simulink model "EcoSIM3_P2_C2_WIP"  (R2014b)
settings: Solver=ode1  SolverMode=SingleTasking  StartTime=0.0  StopTime=4  FixedStep=0.01  RelTol=1e-3
PostLoadFcn:
  | %, if any(exist('dsrtsu_mdlpostloadfcn', 'file') == [2, 3, 6]), try dsrtsu_mdlpostloadfcn('Execute', bdroot); catch fprintf('Error in PostLoadFcn (dsrtsu_mdlpostloadfcn) for model "%s":\n %s\n', bdroot, lasterr); end, end,
InitFcn:
  | tic
  | %Startup_EcoSIM
undefined symbols (not defined in the file or in its folder): canChannel, Controls, DriveCycles, Driver, EM_EFF_MAP, EM_PwrLoss_MAP, EngPwr, EngSpd, EngTrq, Glbl, Overwritten_Mode, Plants, Power, sigbuilder_block, Torque, Trialmap, Veh_Dynamics
libraries: simulink x135, canmsglib x113, fl_lib x104, canlib x89, nesl_utility x56, sdl_lib x29, dspsigops x6, dspswit3 x5, dspstat3 x2, commnoisgen2 x1, dspfdesign x1
(part 17 of 21)

== system EcoSIM3_P2_C2_WIP/Powertrain/Soft_ECUs_IO/VNT Kvaser/CANTx/GMLAN/PPEI_Brake_Apply_Status ==
  GM : Inport
  Bus Selector3 : BusSelector  OutputSignals=PPEI_Brake_Apply_Status.BrkPdlPos
  CAN Pack1 : canmsglib/CAN Pack  CANdbFile=C:\Users\EcoCAR_HIL\Documents\Khanna\EcoSIM3_P1_0_PHEV_TCU\Final_DBC\GlobalAHS_anon GM CONFIDENTIAL.dbc  MsgList=PPEI_Brake_Apply_Status  MsgName=PPEI_Brake_Apply_Status  MsgIDType=Standard (11-bit identifier)  MsgIdentifier=241  MsgLength=6  SignalInfo=BrkAppSnsrHmPosLrnd$30$1$2$2$1$0$1$0$0$1$#BrkPdlChkData$40$17$2$2$1$0$1$0$0$131071$#BrkPdlInTrvPrt$2$2$2$2$1$0$1$0$0$3$#BrkPdlModTrvl$6$1$2$2$1$0$1$0$0$1$#BrkPdlModTrvlV$7$1$2$2$1$0$1$0$0$1$#BrkPdlPos$8$8$2$2$1$0$3.921570e-01$0$0$1.000000e+02$#BrkPdlPosGrad$16$8$2$1$1$0$40$0$-5120$5080$#BrkPedPosAlvRolngCnt$4$2$2$2$1$0$1$0$0$3$#BrkPedTrvlAchvd$1$1$2$2$1$0$1$0$0$1$#BrkPedTrvlAchvdV$0$1$2$2$1$0$1$0$0$1$#NotEventStat$28$2$2$2$1$0$1$0$0$3$#  NSignals=11  StartBits=str2num('[int32(30);int32(40);int32(2);int32(6);int32(7);int32(8);int32(16);int32(4);int32(1);int32(0);int32(28)]')  SignalSizes=str2num('[int32(1);int32(17);int32(2);int32(1);int32(1);int32(8);int32(8);int32(2);int32(1);int32(1);int32(2)]')  ByteOrders=str2num('[int32(2);int32(2);int32(2);int32(2);int32(2);int32(2);int32(2);int32(2);int32(2);int32(2);int32(2)]')  DataTypes=str2num('[int32(2);int32(2);int32(2);int32(2);int32(2);int32(2);int32(1);int32(2);int32(2);int32(2);int32(2)]')  MultiplexTypes=str2num('[int32(1);int32(1);int32(1);int32(1);int32(1);int32(1);int32(1);int32(1);int32(1);int32(1);int32(1)]')  MultiplexValues=str2num('[double(0);double(0);double(0);double(0);double(0);double(0);double(0);double(0);double(0);double(0);double(0)]')  Factors=str2num('[double(1);double(1);double(1);double(1);double(1);double(3.921570e-01);double(40);double(1);double(1);double(1);double(1)]')  Offsets=str2num('[double(0);double(0);double(0);double(0);double(0);double(0);double(0);double(0);double(0);double(0);double(0)]')  Minimums=str2num('[double(0);double(0);double(0);double(0);double(0);double(0);double(-5120);double(0);double(0);double(0);double(0)]')  Maximums=str2num('[double(1);double(131071);double(3);double(1);double(1);double(1.000000e+02);double(5080);double(3);double(1);double(1);double(3)]')  Remote=off
      settings: DataFormat=CANdb specified signals
  CAN Transmit2 : canlib/CAN Transmit  BlockHandle=3142.0018  DeviceMenu=Kvaser Virtual 1 (Channel 1)  Device=Kvaser Virtual 1 (Channel 1)  ObjConstructor=canChannel('Kvaser', 'Virtual 1', 1)  EnablePeriodicTransmit=off  MessagePeriod=1.000
  Ground_{1..10} (10 alike) : Ground
  Rate Transition : RateTransition
  wires:
  Ground_1/1 -> CAN Pack1/1
  Ground_5/1 -> CAN Pack1/5
  Ground_4/1 -> CAN Pack1/4
  Ground_6/1 -> CAN Pack1/7
  Ground_2/1 -> CAN Pack1/2
  Ground_3/1 -> CAN Pack1/3
  Ground_10/1 -> CAN Pack1/11
  Ground_7/1 -> CAN Pack1/8
  Ground_8/1 -> CAN Pack1/9
  Ground_9/1 -> CAN Pack1/10
  Bus Selector3/1 -> Rate Transition/1  "<BrkPdlPos>"
  GM/1 -> Bus Selector3/1
  Rate Transition/1 -> CAN Pack1/6
  CAN Pack1/1 -> CAN Transmit2/1

== system EcoSIM3_P2_C2_WIP/Powertrain/Soft_ECUs_IO/VNT Kvaser/CANTx/GMLAN/PPEI_Driven_Whl_Rotational_Stat ==
  GM : Inport
  Bus Selector2 : BusSelector  OutputSignals=PPEI_Driven_Whl_Rotational_Stat.WRSLDWhlDistPlsCntr,PPEI_Driven_Whl_Rotational_Stat.WRSRDWhlDistPlsCntr
  CAN Pack4 : canmsglib/CAN Pack  CANdbFile=C:\Users\EcoCAR_HIL\Documents\Khanna\EcoSIM3_P1_0_PHEV_TCU\Final_DBC\GlobalAHS_anon GM CONFIDENTIAL.dbc  MsgList=PPEI_Driven_Whl_Rotational_Stat  MsgName=PPEI_Driven_Whl_Rotational_Stat  MsgIDType=Standard (11-bit identifier)  MsgIdentifier=193  MsgLength=8  SignalInfo=WRSLDSeqNum$4$2$2$2$1$0$1$0$0$3$#WRSLDWhlDisTpRC$6$2$2$2$1$0$1$0$0$3$#WRSLDWhlDistPlsCntr$8$10$2$2$1$0$1$0$0$1023$#WRSLDWhlDistTmstm$24$16$2$2$1$0$1$0$0$65535$#WRSLDWhlDistVal$2$1$2$2$1$0$1$0$0$1$#WRSLDWhlRotStatRst$3$1$2$2$1$0$1$0$0$1$#WRSRDSeqNum$36$2$2$2$1$0$1$0$0$3$#WRSRDWhlDisTpRC$38$2$2$2$1$0$1$0$0$3$#WRSRDWhlDistPlsCntr$40$10$2$2$1$0$1$0$0$1023$#WRSRDWhlDistTmstm$56$16$2$2$1$0$1$0$0$65535$#WRSRDWhlDistVal$34$1$2$2$1$0$1$0$0$1$#WRSRDWhlRotStatRst$35$1$2$2$1$0$1$0$0$1$#  NSignals=12  StartBits=str2num('[int32(4);int32(6);int32(8);int32(24);int32(2);int32(3);int32(36);int32(38);int32(40);int32(56);int32(34);int32(35)]')  SignalSizes=str2num('[int32(2);int32(2);int32(10);int32(16);int32(1);int32(1);int32(2);int32(2);int32(10);int32(16);int32(1);int32(1)]')  ByteOrders=str2num('[int32(2);int32(2);int32(2);int32(2);int32(2);int32(2);int32(2);int32(2);int32(2);int32(2);int32(2);int32(2)]')  DataTypes=str2num('[int32(2);int32(2);int32(2);int32(2);int32(2);int32(2);int32(2);int32(2);int32(2);int32(2);int32(2);int32(2)]')  MultiplexTypes=str2num('[int32(1);int32(1);int32(1);int32(1);int32(1);int32(1);int32(1);int32(1);int32(1);int32(1);int32(1);int32(1)]')  MultiplexValues=str2num('[double(0);double(0);double(0);double(0);double(0);double(0);double(0);double(0);double(0);double(0);double(0);double(0)]')  Factors=str2num('[double(1);double(1);double(1);double(1);double(1);double(1);double(1);double(1);double(1);double(1);double(1);double(1)]')  Offsets=str2num('[double(0);double(0);double(0);double(0);double(0);double(0);double(0);double(0);double(0);double(0);double(0);double(0)]')  Minimums=str2num('[double(0);double(0);double(0);double(0);double(0);double(0);double(0);double(0);double(0);double(0);double(0);double(0)]')  Maximums=str2num('[double(3);double(3);double(1023);double(65535);double(1);double(1);double(3);double(3);double(1023);double(65535);double(1);double(1)]')  Remote=off
      settings: DataFormat=CANdb specified signals
  CAN Transmit2 : canlib/CAN Transmit  BlockHandle=3172.0018  DeviceMenu=Kvaser Virtual 1 (Channel 1)  Device=Kvaser Virtual 1 (Channel 1)  ObjConstructor=canChannel('Kvaser', 'Virtual 1', 1)  EnablePeriodicTransmit=off  MessagePeriod=1.000
  Ground_{50..59} (10 alike) : Ground
  Rate Transition : RateTransition
  Rate Transition1 : RateTransition
  wires:
  Bus Selector2/1 -> Rate Transition/1  "<WRSLDWhlDistPlsCntr>"
  Bus Selector2/2 -> Rate Transition1/1  "<WRSRDWhlDistPlsCntr>"
  Ground_57/1 -> CAN Pack4/10
  Ground_50/1 -> CAN Pack4/1
  Ground_59/1 -> CAN Pack4/12
  Ground_53/1 -> CAN Pack4/5
  Ground_52/1 -> CAN Pack4/4
  Ground_51/1 -> CAN Pack4/2
  Ground_54/1 -> CAN Pack4/6
  Ground_55/1 -> CAN Pack4/7
  Ground_56/1 -> CAN Pack4/8
  Ground_58/1 -> CAN Pack4/11
  GM/1 -> Bus Selector2/1
  Rate Transition/1 -> CAN Pack4/3
  Rate Transition1/1 -> CAN Pack4/9
  CAN Pack4/1 -> CAN Transmit2/1

== system EcoSIM3_P2_C2_WIP/Powertrain/Soft_ECUs_IO/VNT Kvaser/CANTx/GMLAN/PPEI_NonDrivn_Whl_Rotationl_Stat ==
  GM : Inport
  Bus Selector5 : BusSelector  OutputSignals=PPEI_NonDrivn_Whl_Rotationl_Stat.WRSLNDWhlDistPCntr,PPEI_NonDrivn_Whl_Rotationl_Stat.WRSRNDWhlDistPCntr
  CAN Pack5 : canmsglib/CAN Pack  CANdbFile=C:\Users\EcoCAR_HIL\Documents\Khanna\EcoSIM3_P1_0_PHEV_TCU\Final_DBC\GlobalAHS_anon GM CONFIDENTIAL.dbc  MsgList=PPEI_NonDrivn_Whl_Rotationl_Stat  MsgName=PPEI_NonDrivn_Whl_Rotationl_Stat  MsgIDType=Standard (11-bit identifier)  MsgIdentifier=197  MsgLength=8  SignalInfo=WRSLNDSeqNum$4$2$2$2$1$0$1$0$0$3$#WRSLNDWhlDisTpRC$6$2$2$2$1$0$1$0$0$3$#WRSLNDWhlDistPCntr$8$10$2$2$1$0$1$0$0$1023$#WRSLNDWhlDistTstm$24$16$2$2$1$0$1$0$0$65535$#WRSLNDWhlDistVal$2$1$2$2$1$0$1$0$0$1$#WRSLNDWhlRotStRst$3$1$2$2$1$0$1$0$0$1$#WRSRNDSeqNum$36$2$2$2$1$0$1$0$0$3$#WRSRNDWhlDisTpRC$38$2$2$2$1$0$1$0$0$3$#WRSRNDWhlDistPCntr$40$10$2$2$1$0$1$0$0$1023$#WRSRNDWhlDistTstm$56$16$2$2$1$0$1$0$0$65535$#WRSRNDWhlDistVal$34$1$2$2$1$0$1$0$0$1$#WRSRNDWhlRotStRst$35$1$2$2$1$0$1$0$0$1$#  NSignals=12  StartBits=str2num('[int32(4);int32(6);int32(8);int32(24);int32(2);int32(3);int32(36);int32(38);int32(40);int32(56);int32(34);int32(35)]')  SignalSizes=str2num('[int32(2);int32(2);int32(10);int32(16);int32(1);int32(1);int32(2);int32(2);int32(10);int32(16);int32(1);int32(1)]')  ByteOrders=str2num('[int32(2);int32(2);int32(2);int32(2);int32(2);int32(2);int32(2);int32(2);int32(2);int32(2);int32(2);int32(2)]')  DataTypes=str2num('[int32(2);int32(2);int32(2);int32(2);int32(2);int32(2);int32(2);int32(2);int32(2);int32(2);int32(2);int32(2)]')  MultiplexTypes=str2num('[int32(1);int32(1);int32(1);int32(1);int32(1);int32(1);int32(1);int32(1);int32(1);int32(1);int32(1);int32(1)]')  MultiplexValues=str2num('[double(0);double(0);double(0);double(0);double(0);double(0);double(0);double(0);double(0);double(0);double(0);double(0)]')  Factors=str2num('[double(1);double(1);double(1);double(1);double(1);double(1);double(1);double(1);double(1);double(1);double(1);double(1)]')  Offsets=str2num('[double(0);double(0);double(0);double(0);double(0);double(0);double(0);double(0);double(0);double(0);double(0);double(0)]')  Minimums=str2num('[double(0);double(0);double(0);double(0);double(0);double(0);double(0);double(0);double(0);double(0);double(0);double(0)]')  Maximums=str2num('[double(3);double(3);double(1023);double(65535);double(1);double(1);double(3);double(3);double(1023);double(65535);double(1);double(1)]')  Remote=off
      settings: DataFormat=CANdb specified signals
  CAN Transmit2 : canlib/CAN Transmit  BlockHandle=3205.0018  DeviceMenu=Kvaser Virtual 1 (Channel 1)  Device=Kvaser Virtual 1 (Channel 1)  ObjConstructor=canChannel('Kvaser', 'Virtual 1', 1)  EnablePeriodicTransmit=off  MessagePeriod=1.000
  Ground_{60..69} (10 alike) : Ground
  Rate Transition : RateTransition
  Rate Transition1 : RateTransition
  wires:
  Bus Selector5/2 -> Rate Transition1/1  "<WRSRNDWhlDistPCntr>"
  Bus Selector5/1 -> Rate Transition/1  "<WRSLNDWhlDistPCntr>"
  Ground_60/1 -> CAN Pack5/1
  Ground_69/1 -> CAN Pack5/12
  Ground_63/1 -> CAN Pack5/5
  Ground_61/1 -> CAN Pack5/2
  Ground_66/1 -> CAN Pack5/8
  Ground_67/1 -> CAN Pack5/10
  Ground_68/1 -> CAN Pack5/11
  Ground_65/1 -> CAN Pack5/7
  Ground_64/1 -> CAN Pack5/6
  Ground_62/1 -> CAN Pack5/4
  GM/1 -> Bus Selector5/1
  Rate Transition/1 -> CAN Pack5/3
  Rate Transition1/1 -> CAN Pack5/9
  CAN Pack5/1 -> CAN Transmit2/1

== system EcoSIM3_P2_C2_WIP/Powertrain/Soft_ECUs_IO/VNT Kvaser/CANTx/GMLAN/PPEI_Platform_General_Status ==
  GM : Inport
  Bus Selector1 : BusSelector  OutputSignals=PPEI_Platform_General_Status.SysPwrMd
  CAN Pack2 : canmsglib/CAN Pack  CANdbFile=C:\Users\EcoCAR_HIL\Documents\Khanna\EcoSIM3_P1_0_PHEV_TCU\Final_DBC\GlobalAHS_anon GM CONFIDENTIAL.dbc  MsgList=PPEI_Platform_General_Status  MsgName=PPEI_Platform_General_Status  MsgIDType=Standard (11-bit identifier)  MsgIdentifier=497  MsgLength=8  SignalInfo=ACCmpsrFldOn$63$1$2$2$1$0$1$0$0$1$#ACCompModReq$11$2$2$2$1$0$1$0$0$3$#ACCompNormLd$48$8$2$2$1$0$1.000000e-01$0$0$2.550000e+01$#ACCompNormLdV$10$1$2$2$1$0$1$0$0$1$#ACCompSysVDA$9$1$2$2$1$0$1$0$0$1$#ACCompSysVDM$60$1$2$2$1$0$1$0$0$1$#AirbgVDA$57$1$2$2$1$0$1$0$0$1$#BkupPwrModeMstrVDA$7$1$2$2$1$0$1$0$0$1$#BkupPwrModeMstrVDM$61$1$2$2$1$0$1$0$0$1$#DispMeasSys$59$1$2$2$1$0$1$0$0$1$#ElvtdIdlCstStReq$32$2$2$2$1$0$1$0$0$3$#EngOilLfRstRq$37$1$2$2$1$0$1$0$0$1$#FuelFltLfRstRqd$56$1$2$2$1$0$1$0$0$1$#ImmblzrPreRelPswdStat$8$1$2$2$1$0$1$0$0$1$#ImmblzrPreRelPswrd$24$16$2$2$1$0$1$0$0$65535$#PMMAccTrmSt$2$1$2$2$1$0$1$0$0$1$#PMMRunCrkTrmSt$3$1$2$2$1$0$1$0$0$1$#PTORSMstrEngShtReq$13$1$2$2$1$0$1$0$0$1$#PTORmStMsEngStRq$14$1$2$2$1$0$1$0$0$1$#PrkBrkSwAtv$36$1$2$2$1$0$1$0$0$1$#PrkBrkVDA$35$1$2$2$1$0$1$0$0$1$#PrkBrkVDM$62$1$2$2$1$0$1$0$0$1$#RmVehStrRq$15$1$2$2$1$0$1$0$0$1$#SIRDpl$58$1$2$2$1$0$1$0$0$1$#SysBkUpPwrMd$4$2$2$2$1$0$1$0$0$3$#SysBkupPwrMdEn$6$1$2$2$1$0$1$0$0$1$#SysPwrMd$0$2$2$2$1$0$1$0$0$3$#ThrtlPrgrsnReq$38$2$2$2$1$0$1$0$0$3$#TrStLgMdAtv$34$1$2$2$1$0$1$0$0$1$#  NSignals=29  StartBits=str2num('[int32(63);int32(11);int32(48);int32(10);int32(9);int32(60);int32(57);int32(7);int32(61);int32(59);int32(32);int32(37);int32(56);int32(8);int32(24);int32(2);int32(3);int32(13);int32(14);int32(36);int32(35);int32(62);int32(15);int32(58);int32(4);int32(6);int32(0);int32(38);int32(34)]')  SignalSizes=str2num('[int32(1);int32(2);int32(8);int32(1);int32(1);int32(1);int32(1);int32(1);int32(1);int32(1);int32(2);int32(1);int32(1);int32(1);int32(16);int32(1);int32(1);int32(1);int32(1);int32(1);int32(1);int32(1);int32(1);int32(1);int32(2);int32(1);int32(2);int32(2);int32(1)]')  ByteOrders=str2num('[int32(2);int32(2);int32(2);int32(2);int32(2);int32(2);int32(2);int32(2);int32(2);int32(2);int32(2);int32(2);int32(2);int32(2);int32(2);int32(2);int32(2);int32(2);int32(2);int32(2);int32(2);int32(2);int32(2);int32(2);int32(2);int32(2);int32(2);int32(2);int32(2)]')  DataTypes=str2num('[int32(2);int32(2);int32(2);int32(2);int32(2);int32(2);int32(2);int32(2);int32(2);int32(2);int32(2);int32(2);int32(2);int32(2);int32(2);int32(2);int32(2);int32(2);int32(2);int32(2);int32(2);int32(2);int32(2);int32(2);int32(2);int32(2);int32(2);int32(2);int32(2)]')  MultiplexTypes=str2num('[int32(1);int32(1);int32(1);int32(1);int32(1);int32(1);int32(1);int32(1);int32(1);int32(1);int32(1);int32(1);int32(1);int32(1);int32(1);int32(1);int32(1);int32(1);int32(1);int32(1);int32(1);int32(1);int32(1);int32(1);int32(1);int32(1);int32(1);int32(1);int32(1)]')  MultiplexValues=str2num('[double(0);double(0);double(0);double(0);double(0);double(0);double(0);double(0);double(0);double(0);double(0);double(0);double(0);double(0);double(0);double(0);double(0);double(0);double(0);double(0);double(0);double(0);double(0);double(0);double(0);double(0);double(0);double(0);double(0)]')  Factors=str2num('[double(1);double(1);double(1.000000e-01);double(1);double(1);double(1);double(1);double(1);double(1);double(1);double(1);double(1);double(1);double(1);double(1);double(1);double(1);double(1);double(1);double(1);double(1);double(1);double(1);double(1);double(1);double(1);double(1);double(1);double(1)]')  Offsets=str2num('[double(0);double(0);double(0);double(0);double(0);double(0);double(0);double(0);double(0);double(0);double(0);double(0);double(0);double(0);double(0);double(0);double(0);double(0);double(0);double(0);double(0);double(0);double(0);double(0);double(0);double(0);double(0);double(0);double(0)]')  Minimums=str2num('[double(0);double(0);double(0);double(0);double(0);double(0);double(0);double(0);double(0);double(0);double(0);double(0);double(0);double(0);double(0);double(0);double(0);double(0);double(0);double(0);double(0);double(0);double(0);double(0);double(0);double(0);double(0);double(0);double(0)]')  Maximums=str2num('[double(1);double(3);double(2.550000e+01);double(1);double(1);double(1);double(1);double(1);double(1);double(1);double(3);double(1);double(1);double(1);double(65535);double(1);double(1);double(1);double(1);double(1);double(1);double(1);double(1);double(1);double(3);double(1);double(3);double(3);double(1)]')  Remote=off
      settings: DataFormat=CANdb specified signals
  CAN Transmit2 : canlib/CAN Transmit  BlockHandle=3238.0018  DeviceMenu=Kvaser Virtual 1 (Channel 1)  Device=Kvaser Virtual 1 (Channel 1)  ObjConstructor=canChannel('Kvaser', 'Virtual 1', 1)  EnablePeriodicTransmit=off  MessagePeriod=1.000
  Ground_{11..38} (28 alike) : Ground
  Rate Transition : RateTransition
  wires:
  Ground_29/1 -> CAN Pack2/19
  Ground_32/1 -> CAN Pack2/22
  Ground_35/1 -> CAN Pack2/25
  Ground_11/1 -> CAN Pack2/1
  Ground_27/1 -> CAN Pack2/17
  Ground_15/1 -> CAN Pack2/5
  Ground_37/1 -> CAN Pack2/28
  Ground_13/1 -> CAN Pack2/3
  Ground_16/1 -> CAN Pack2/6
  Ground_24/1 -> CAN Pack2/14
  Ground_25/1 -> CAN Pack2/15
  Ground_14/1 -> CAN Pack2/4
  Ground_28/1 -> CAN Pack2/18
  Ground_31/1 -> CAN Pack2/21
  Ground_38/1 -> CAN Pack2/29
  Ground_21/1 -> CAN Pack2/11
  Ground_26/1 -> CAN Pack2/16
  Ground_30/1 -> CAN Pack2/20
  Ground_20/1 -> CAN Pack2/10
  Ground_17/1 -> CAN Pack2/7
  Ground_22/1 -> CAN Pack2/12
  Ground_36/1 -> CAN Pack2/26
  Ground_33/1 -> CAN Pack2/23
  Ground_18/1 -> CAN Pack2/8
  Ground_34/1 -> CAN Pack2/24
  Ground_12/1 -> CAN Pack2/2
  Ground_19/1 -> CAN Pack2/9
  Ground_23/1 -> CAN Pack2/13
  Bus Selector1/1 -> Rate Transition/1  "<SysPwrMd>"
  GM/1 -> Bus Selector1/1
  Rate Transition/1 -> CAN Pack2/27
  CAN Pack2/1 -> CAN Transmit2/1

== system EcoSIM3_P2_C2_WIP/Powertrain/Soft_ECUs_IO/VNT Kvaser/CANTx/GMLAN/PPEI_Vehicle_Speed_and_Distance ==
  GM : Inport
  Bus Selector4 : BusSelector  OutputSignals=PPEI_Vehicle_Speed_and_Distance.VehSpdAvgDrvn
  CAN Pack3 : canmsglib/CAN Pack  CANdbFile=C:\Users\EcoCAR_HIL\Documents\Khanna\EcoSIM3_P1_0_PHEV_TCU\Final_DBC\GlobalAHS_anon GM CONFIDENTIAL.dbc  MsgList=PPEI_Vehicle_Speed_and_Distance  MsgName=PPEI_Vehicle_Speed_and_Distance  MsgIDType=Standard (11-bit identifier)  MsgIdentifier=1001  MsgLength=8  SignalInfo=DistRollCntAvgDrvn$24$13$2$2$1$0$1.250000e-01$0$0$1.023875e+03$#DistRollCntAvgDrvnSrc$55$1$2$2$1$0$1$0$0$1$#DistRollCntAvgDrvnV$22$1$2$2$1$0$1$0$0$1$#DstRolCntAvNDrRstOc$53$1$2$2$1$0$1$0$0$1$#DstRolCntAvgDrnRstOc$21$1$2$2$1$0$1$0$0$1$#DstRolCntAvgNonDrvn$56$13$2$2$1$0$1.250000e-01$0$0$1.023875e+03$#DstRolCntAvgNonDrvnV$54$1$2$2$1$0$1$0$0$1$#VehSpdAvgDrvn$8$15$2$2$1$0$1.562500e-02$0$0$5.119844e+02$#VehSpdAvgDrvnSrc$23$1$2$2$1$0$1$0$0$1$#VehSpdAvgDrvnV$7$1$2$2$1$0$1$0$0$1$#VehSpdAvgNDrvn$40$15$2$2$1$0$1.562500e-02$0$0$5.119844e+02$#VehSpdAvgNDrvnV$39$1$2$2$1$0$1$0$0$1$#  NSignals=12  StartBits=str2num('[int32(24);int32(55);int32(22);int32(53);int32(21);int32(56);int32(54);int32(8);int32(23);int32(7);int32(40);int32(39)]')  SignalSizes=str2num('[int32(13);int32(1);int32(1);int32(1);int32(1);int32(13);int32(1);int32(15);int32(1);int32(1);int32(15);int32(1)]')  ByteOrders=str2num('[int32(2);int32(2);int32(2);int32(2);int32(2);int32(2);int32(2);int32(2);int32(2);int32(2);int32(2);int32(2)]')  DataTypes=str2num('[int32(2);int32(2);int32(2);int32(2);int32(2);int32(2);int32(2);int32(2);int32(2);int32(2);int32(2);int32(2)]')  MultiplexTypes=str2num('[int32(1);int32(1);int32(1);int32(1);int32(1);int32(1);int32(1);int32(1);int32(1);int32(1);int32(1);int32(1)]')  MultiplexValues=str2num('[double(0);double(0);double(0);double(0);double(0);double(0);double(0);double(0);double(0);double(0);double(0);double(0)]')  Factors=str2num('[double(1.250000e-01);double(1);double(1);double(1);double(1);double(1.250000e-01);double(1);double(1.562500e-02);double(1);double(1);double(1.562500e-02);double(1)]')  Offsets=str2num('[double(0);double(0);double(0);double(0);double(0);double(0);double(0);double(0);double(0);double(0);double(0);double(0)]')  Minimums=str2num('[double(0);double(0);double(0);double(0);double(0);double(0);double(0);double(0);double(0);double(0);double(0);double(0)]')  Maximums=str2num('[double(1.023875e+03);double(1);double(1);double(1);double(1);double(1.023875e+03);double(1);double(5.119844e+02);double(1);double(1);double(5.119844e+02);double(1)]')  Remote=off
      settings: DataFormat=CANdb specified signals
  CAN Transmit2 : canlib/CAN Transmit  BlockHandle=3304.0018  DeviceMenu=Kvaser Virtual 1 (Channel 1)  Device=Kvaser Virtual 1 (Channel 1)  ObjConstructor=canChannel('Kvaser', 'Virtual 1', 1)  EnablePeriodicTransmit=off  MessagePeriod=1.000
  Ground_{39..49} (11 alike) : Ground
  Rate Transition : RateTransition
  wires:
  Ground_47/1 -> CAN Pack3/10
  Ground_45/1 -> CAN Pack3/7
  Ground_44/1 -> CAN Pack3/6
  Ground_46/1 -> CAN Pack3/9
  Ground_49/1 -> CAN Pack3/12
  Ground_48/1 -> CAN Pack3/11
  Ground_42/1 -> CAN Pack3/4
  Ground_40/1 -> CAN Pack3/2
  Ground_39/1 -> CAN Pack3/1
  Ground_43/1 -> CAN Pack3/5
  Ground_41/1 -> CAN Pack3/3
  Bus Selector4/1 -> Rate Transition/1  "<VehSpdAvgDrvn>"
  GM/1 -> Bus Selector4/1
  Rate Transition/1 -> CAN Pack3/8
  CAN Pack3/1 -> CAN Transmit2/1

== system EcoSIM3_P2_C2_WIP/Powertrain/Soft_ECUs_IO/VNT Vector/CANTx/BAS/Status_1 ==
  In1 : Inport
  Bus Selector5 : BusSelector  OutputSignals=Status_1.BAS_Speed_rad_per_s,Status_1.BAS_Torque_Out_Nm
  CAN Pack5 : canmsglib/CAN Pack  CANdbFile=C:\Box Sync\EcoCAR 3\SMS\EcoSIM3_P2_C2\MIL\Final_DBC\InfineonInverter.dbc  MsgList=Status_1  MsgName=Status_1  MsgIDType=Standard (11-bit identifier)  MsgIdentifier=257  MsgLength=8  SignalInfo=Checksum3$0$8$1$2$1$0$1$0$-Inf$Inf$#CoolingReq$55$1$1$2$1$0$1$0$0$1$#Counter3$8$8$1$2$1$0$1$0$0$15$#ErrorInfo$48$2$1$2$1$0$1$0$0$3$#PowerRed$50$4$1$2$1$0$1$0$0$15$#ReadyHV$54$1$1$2$1$0$1$0$0$1$#RegAtLimit$56$1$1$2$1$0$1$0$0$1$#Reserved4$59$1$1$2$1$0$1$0$0$1$#SetLimitsOk$57$1$1$2$1$0$1$0$0$1$#SetValuesOk$58$1$1$2$1$0$1$0$0$1$#Speed$32$16$1$1$1$0$5.000000e-01$0$-16384$1.638350e+04$#StatusMode$60$4$1$2$1$0$1$0$0$15$#Torque_Normalized$16$16$1$1$1$0$3.051758e-05$0$-1$9.999695e-01$#  NSignals=13  StartBits=str2num('[int32(0);int32(55);int32(8);int32(48);int32(50);int32(54);int32(56);int32(59);int32(57);int32(58);int32(32);int32(60);int32(16)]')  SignalSizes=str2num('[int32(8);int32(1);int32(8);int32(2);int32(4);int32(1);int32(1);int32(1);int32(1);int32(1);int32(16);int32(4);int32(16)]')  ByteOrders=str2num('[int32(1);int32(1);int32(1);int32(1);int32(1);int32(1);int32(1);int32(1);int32(1);int32(1);int32(1);int32(1);int32(1)]')  DataTypes=str2num('[int32(2);int32(2);int32(2);int32(2);int32(2);int32(2);int32(2);int32(2);int32(2);int32(2);int32(1);int32(2);int32(1)]')  MultiplexTypes=str2num('[int32(1);int32(1);int32(1);int32(1);int32(1);int32(1);int32(1);int32(1);int32(1);int32(1);int32(1);int32(1);int32(1)]')  MultiplexValues=str2num('[double(0);double(0);double(0);double(0);double(0);double(0);double(0);double(0);double(0);double(0);double(0);double(0);double(0)]')  Factors=str2num('[double(1);double(1);double(1);double(1);double(1);double(1);double(1);double(1);double(1);double(1);double(5.000000e-01);double(1);double(3.051758e-05)]')  Offsets=str2num('[double(0);double(0);double(0);double(0);double(0);double(0);double(0);double(0);double(0);double(0);double(0);double(0);double(0)]')  Minimums=str2num('[double(-Inf);double(0);double(0);double(0);double(0);double(0);double(0);double(0);double(0);double(0);double(-16384);double(0);double(-1)]')  Maximums=str2num('[double(Inf);double(1);double(15);double(3);double(15);double(1);double(1);double(1);double(1);double(1);double(1.638350e+04);double(15);double(9.999695e-01)]')  Remote=off
      settings: DataFormat=CANdb specified signals
  Ground_{16..26} (11 alike) : Ground
  Rate Transition : RateTransition
  Rate Transition1 : RateTransition
  Out1 : Outport
  wires:
  In1/1 -> Bus Selector5/1
  CAN Pack5/1 -> Out1/1
  Ground_24/1 -> CAN Pack5/9
  Ground_26/1 -> CAN Pack5/12
  Bus Selector5/2 -> Rate Transition1/1  "<BAS_Torque_Out_Nm>"
  Ground_22/1 -> CAN Pack5/7
  Ground_19/1 -> CAN Pack5/4
  Bus Selector5/1 -> Rate Transition/1  "<BAS_Speed_rad_per_s>"
  Ground_23/1 -> CAN Pack5/8
  Ground_18/1 -> CAN Pack5/3
  Ground_20/1 -> CAN Pack5/5
  Ground_21/1 -> CAN Pack5/6
  Ground_25/1 -> CAN Pack5/10
  Ground_17/1 -> CAN Pack5/2
  Ground_16/1 -> CAN Pack5/1
  Rate Transition/1 -> CAN Pack5/11
  Rate Transition1/1 -> CAN Pack5/13

== system EcoSIM3_P2_C2_WIP/Powertrain/Soft_ECUs_IO/VNT Vector/CANTx/BAS/Status_2 ==
  In1 : Inport
  Bus Selector1 : BusSelector  OutputSignals=Status_2.Fault_U,Status_2.Fault_V,Status_2.Fault_W
  CAN Pack1 : canmsglib/CAN Pack  CANdbFile=C:\Box Sync\EcoCAR 3\SMS\EcoSIM3_P2_C2\MIL\Final_DBC\InfineonInverter.dbc  MsgList=Status_2  MsgName=Status_2  MsgIDType=Standard (11-bit identifier)  MsgIdentifier=273  MsgLength=8  SignalInfo=Checksum4$0$8$1$2$1$0$1$0$-Inf$Inf$#Counter4$8$4$1$2$1$0$1$0$0$15$#CurrentD_Limit$32$16$1$1$3$7$3.125000e-02$0$-1024$1.023969e+03$#CurrentD_Reference$32$16$1$1$3$9$3.125000e-02$0$-1024$1.023969e+03$#CurrentQ_Limit$32$16$1$1$3$6$3.125000e-02$0$-1024$1.023969e+03$#CurrentQ_Reference$32$16$1$1$3$8$3.125000e-02$0$-1024$1.023969e+03$#FaultU$13$1$1$2$1$0$1$0$0$1$#FaultV$14$1$1$2$1$0$1$0$0$1$#FaultW$15$1$1$2$1$0$1$0$0$1$#MultiplexCode$48$16$1$2$2$0$1$0$0$65535$#PhaseU_IGBT_Temp$32$16$1$1$3$3$7.812500e-03$0$-256$2.559922e+02$#PhaseV_IGBT_Temp$32$16$1$1$3$4$7.812500e-03$0$-256$2.559922e+02$#PhaseW_IGBT_Temp$32$16$1$1$3$5$7.812500e-03$0$-256$2.559922e+02$#RehabilitationReq$12$1$1$2$1$0$1$0$0$1$#Software_Version$32$16$1$2$3$0$1$0$0$65535$#Speed_Command$32$16$1$1$3$1$5.000000e-01$0$-16384$1.638350e+04$#Stator_Temperature$32$16$1$1$3$2$7.812500e-03$0$-256$2.559922e+02$#VoltageDC$16$16$1$1$1$0$3.125000e-02$0$-1024$1.023969e+03$#  NSignals=18  StartBits=str2num('[int32(0);int32(8);int32(32);int32(32);int32(32);int32(32);int32(13);int32(14);int32(15);int32(48);int32(32);int32(32);int32(32);int32(12);int32(32);int32(32);int32(32);int32(16)]')  SignalSizes=str2num('[int32(8);int32(4);int32(16);int32(16);int32(16);int32(16);int32(1);int32(1);int32(1);int32(16);int32(16);int32(16);int32(16);int32(1);int32(16);int32(16);int32(16);int32(16)]')  ByteOrders=str2num('[int32(1);int32(1);int32(1);int32(1);int32(1);int32(1);int32(1);int32(1);int32(1);int32(1);int32(1);int32(1);int32(1);int32(1);int32(1);int32(1);int32(1);int32(1)]')  DataTypes=str2num('[int32(2);int32(2);int32(1);int32(1);int32(1);int32(1);int32(2);int32(2);int32(2);int32(2);int32(1);int32(1);int32(1);int32(2);int32(2);int32(1);int32(1);int32(1)]')  MultiplexTypes=str2num('[int32(1);int32(1);int32(3);int32(3);int32(3);int32(3);int32(1);int32(1);int32(1);int32(2);int32(3);int32(3);int32(3);int32(1);int32(3);int32(3);int32(3);int32(1)]')  MultiplexValues=str2num('[double(0);double(0);double(7);double(9);double(6);double(8);double(0);double(0);double(0);double(0);double(3);double(4);double(5);double(0);double(0);double(1);double(2);double(0)]')  Factors=str2num('[double(1);double(1);double(3.125000e-02);double(3.125000e-02);double(3.125000e-02);double(3.125000e-02);double(1);double(1);double(1);double(1);double(7.812500e-03);double(7.812500e-03);double(7.812500e-03);double(1);double(1);double(5.000000e-01);double(7.812500e-03);double(3.125000e-02)]')  Offsets=str2num('[double(0);double(0);double(0);double(0);double(0);double(0);double(0);double(0);double(0);double(0);double(0);double(0);double(0);double(0);double(0);double(0);double(0);double(0)]')  Minimums=str2num('[double(-Inf);double(0);double(-1024);double(-1024);double(-1024);double(-1024);double(0);double(0);double(0);double(0);double(-256);double(-256);double(-256);double(0);double(0);double(-16384);double(-256);double(-1024)]')  Maximums=str2num('[double(Inf);double(15);double(1.023969e+03);double(1.023969e+03);double(1.023969e+03);double(1.023969e+03);double(1);double(1);double(1);double(65535);double(2.559922e+02);double(2.559922e+02);double(2.559922e+02);double(1);double(65535);double(1.638350e+04);double(2.559922e+02);double(1.023969e+03)]')  Remote=off
      settings: DataFormat=CANdb specified signals
  Ground_{1..15} (15 alike) : Ground
  Rate Transition1 : RateTransition
  Rate Transition2 : RateTransition
  Rate Transition3 : RateTransition
  Out1 : Outport
  wires:
  Ground_9/1 -> CAN Pack1/12
  Bus Selector1/3 -> Rate Transition3/1  "<Fault_W>"
  Ground_1/1 -> CAN Pack1/1
  Ground_6/1 -> CAN Pack1/6
  In1/1 -> Bus Selector1/1
  CAN Pack1/1 -> Out1/1
  Bus Selector1/2 -> Rate Transition2/1  "<Fault_V>"
  Ground_2/1 -> CAN Pack1/2
  Ground_14/1 -> CAN Pack1/17
  Ground_4/1 -> CAN Pack1/4
  Ground_12/1 -> CAN Pack1/15
  Bus Selector1/1 -> Rate Transition1/1  "<Fault_U>"
  Ground_11/1 -> CAN Pack1/14
  Ground_3/1 -> CAN Pack1/3
  Ground_10/1 -> CAN Pack1/13
  Ground_13/1 -> CAN Pack1/16
  Ground_7/1 -> CAN Pack1/10
  Ground_8/1 -> CAN Pack1/11
  Ground_5/1 -> CAN Pack1/5
  Ground_15/1 -> CAN Pack1/18
  Rate Transition1/1 -> CAN Pack1/7
  Rate Transition2/1 -> CAN Pack1/8
  Rate Transition3/1 -> CAN Pack1/9

== system EcoSIM3_P2_C2_WIP/Powertrain/Soft_ECUs_IO/VNT Vector/CANTx/EM/M160_Temperature_Set_1 ==
  EM : Inport
  Bus Selector5 : BusSelector  OutputSignals=M160_Temperature_Set_1.Module_A,M160_Temperature_Set_1.Module_B,M160_Temperature_Set_1.Module_C,M160_Temperature_Set_1.Gate_Driver_Board
  CAN Pack3 : canmsglib/CAN Pack  CANdbFile=C:\Users\EcoCAR_HIL\Documents\Khanna\EcoSIM3_P1_0_PHEV_TCU\Final_DBC\20160113 RMS PM CAN DB.dbc  MsgList=M160_Temperature_Set_1  MsgName=M160_Temperature_Set_1  MsgIDType=Standard (11-bit identifier)  MsgIdentifier=160  MsgLength=8  SignalInfo=D1_Module_A$0$16$1$1$1$0$1.000000e-01$0$-3.276800e+03$3.276700e+03$#D2_Module_B$16$16$1$1$1$0$1.000000e-01$0$-3.276800e+03$3.276700e+03$#D3_Module_C$32$16$1$1$1$0$1.000000e-01$0$-3.276800e+03$3.276700e+03$#D4_Gate_Driver_Board$48$16$1$1$1$0$1.000000e-01$0$-3.276800e+03$3.276700e+03$#  NSignals=4  StartBits=str2num('[int32(0);int32(16);int32(32);int32(48)]')  SignalSizes=str2num('[int32(16);int32(16);int32(16);int32(16)]')  ByteOrders=str2num('[int32(1);int32(1);int32(1);int32(1)]')  DataTypes=str2num('[int32(1);int32(1);int32(1);int32(1)]')  MultiplexTypes=str2num('[int32(1);int32(1);int32(1);int32(1)]')  MultiplexValues=str2num('[double(0);double(0);double(0);double(0)]')  Factors=str2num('[double(1.000000e-01);double(1.000000e-01);double(1.000000e-01);double(1.000000e-01)]')  Offsets=str2num('[double(0);double(0);double(0);double(0)]')  Minimums=str2num('[double(-3.276800e+03);double(-3.276800e+03);double(-3.276800e+03);double(-3.276800e+03)]')  Maximums=str2num('[double(3.276700e+03);double(3.276700e+03);double(3.276700e+03);double(3.276700e+03)]')  Remote=off
      settings: DataFormat=CANdb specified signals
  Rate Transition{,1..3} (4 alike) : RateTransition
  Out1 : Outport
  wires:
  Bus Selector5/2 -> Rate Transition3/1  "<Module_B>"
  Bus Selector5/4 -> Rate Transition1/1  "<Gate_Driver_Board>"
  Bus Selector5/1 -> Rate Transition/1  "<Module_A>"
  Bus Selector5/3 -> Rate Transition2/1  "<Module_C>"
  EM/1 -> Bus Selector5/1
  Rate Transition/1 -> CAN Pack3/1
  Rate Transition1/1 -> CAN Pack3/4
  Rate Transition2/1 -> CAN Pack3/3
  Rate Transition3/1 -> CAN Pack3/2
  CAN Pack3/1 -> Out1/1

== system EcoSIM3_P2_C2_WIP/Powertrain/Soft_ECUs_IO/VNT Vector/CANTx/EM/M161_Temperature_Set_2 ==
  EM : Inport
  Bus Selector6 : BusSelector  OutputSignals=M161_Temperature_Set_2.Control_Board_Temperature
  CAN Pack5 : canmsglib/CAN Pack  CANdbFile=C:\Users\EcoCAR_HIL\Documents\Khanna\EcoSIM3_P1_0_PHEV_TCU\Final_DBC\20160113 RMS PM CAN DB.dbc  MsgList=M161_Temperature_Set_2  MsgName=M161_Temperature_Set_2  MsgIDType=Standard (11-bit identifier)  MsgIdentifier=161  MsgLength=8  SignalInfo=D1_Control_Board_Temperature$0$16$1$1$1$0$1.000000e-01$0$-3.276800e+03$3.276700e+03$#D2_RTD1_Temperature$16$16$1$1$1$0$1.000000e-01$0$-3.276800e+03$3.276700e+03$#D3_RTD2_Temperature$32$16$1$1$1$0$1.000000e-01$0$-3.276800e+03$3.276700e+03$#D4_RTD3_Temperature$48$16$1$1$1$0$1.000000e-01$0$-3.276800e+03$3.276700e+03$#  NSignals=4  StartBits=str2num('[int32(0);int32(16);int32(32);int32(48)]')  SignalSizes=str2num('[int32(16);int32(16);int32(16);int32(16)]')  ByteOrders=str2num('[int32(1);int32(1);int32(1);int32(1)]')  DataTypes=str2num('[int32(1);int32(1);int32(1);int32(1)]')  MultiplexTypes=str2num('[int32(1);int32(1);int32(1);int32(1)]')  MultiplexValues=str2num('[double(0);double(0);double(0);double(0)]')  Factors=str2num('[double(1.000000e-01);double(1.000000e-01);double(1.000000e-01);double(1.000000e-01)]')  Offsets=str2num('[double(0);double(0);double(0);double(0)]')  Minimums=str2num('[double(-3.276800e+03);double(-3.276800e+03);double(-3.276800e+03);double(-3.276800e+03)]')  Maximums=str2num('[double(3.276700e+03);double(3.276700e+03);double(3.276700e+03);double(3.276700e+03)]')  Remote=off
      settings: DataFormat=CANdb specified signals
  Ground5 : Ground
  Rate Transition : RateTransition
  Out1 : Outport
  wires:
  Bus Selector6/1 -> Rate Transition/1  "<Control_Board_Temperature>"
  Ground5/1 -> CAN Pack5/3, CAN Pack5/2, CAN Pack5/4
  EM/1 -> Bus Selector6/1
  Rate Transition/1 -> CAN Pack5/1
  CAN Pack5/1 -> Out1/1

== system EcoSIM3_P2_C2_WIP/Powertrain/Soft_ECUs_IO/VNT Vector/CANTx/EM/M162_Temperature_Set_3 ==
  EM : Inport
  Bus Selector7 : BusSelector  OutputSignals=M162_Temperature_Set_3.Motor_Temperature
  CAN Pack6 : canmsglib/CAN Pack  CANdbFile=C:\Users\EcoCAR_HIL\Documents\Khanna\EcoSIM3_P1_0_PHEV_TCU\Final_DBC\20160113 RMS PM CAN DB.dbc  MsgList=M162_Temperature_Set_3  MsgName=M162_Temperature_Set_3  MsgIDType=Standard (11-bit identifier)  MsgIdentifier=162  MsgLength=8  SignalInfo=D1_RTD4_Temperature$0$16$1$1$1$0$1.000000e-01$0$-3.276800e+03$3.276700e+03$#D2_RTD5_Temperature$16$16$1$1$1$0$1.000000e-01$0$-3.276800e+03$3.276700e+03$#D3_Motor_Temperature$32$16$1$1$1$0$1.000000e-01$0$-3.276800e+03$3.276700e+03$#D4_Torque_Shudder$48$16$1$1$1$0$1.000000e-01$0$-3.276800e+03$3.276700e+03$#  NSignals=4  StartBits=str2num('[int32(0);int32(16);int32(32);int32(48)]')  SignalSizes=str2num('[int32(16);int32(16);int32(16);int32(16)]')  ByteOrders=str2num('[int32(1);int32(1);int32(1);int32(1)]')  DataTypes=str2num('[int32(1);int32(1);int32(1);int32(1)]')  MultiplexTypes=str2num('[int32(1);int32(1);int32(1);int32(1)]')  MultiplexValues=str2num('[double(0);double(0);double(0);double(0)]')  Factors=str2num('[double(1.000000e-01);double(1.000000e-01);double(1.000000e-01);double(1.000000e-01)]')  Offsets=str2num('[double(0);double(0);double(0);double(0)]')  Minimums=str2num('[double(-3.276800e+03);double(-3.276800e+03);double(-3.276800e+03);double(-3.276800e+03)]')  Maximums=str2num('[double(3.276700e+03);double(3.276700e+03);double(3.276700e+03);double(3.276700e+03)]')  Remote=off
      settings: DataFormat=CANdb specified signals
  Ground6 : Ground
  Rate Transition : RateTransition
  Out1 : Outport
  wires:
  Ground6/1 -> CAN Pack6/1, CAN Pack6/2, CAN Pack6/4
  Bus Selector7/1 -> Rate Transition/1  "<Motor_Temperature>"
  EM/1 -> Bus Selector7/1
  Rate Transition/1 -> CAN Pack6/3
  CAN Pack6/1 -> Out1/1

== system EcoSIM3_P2_C2_WIP/Powertrain/Soft_ECUs_IO/VNT Vector/CANTx/EM/M165_Motor_Position_Info ==
  EM : Inport
  Bus Selector1 : BusSelector  OutputSignals=M165_Motor_Position_Info.Motor_Speed
  CAN Pack1 : canmsglib/CAN Pack  CANdbFile=C:\Users\EcoCAR_HIL\Documents\Khanna\EcoSIM3_P1_0_PHEV_TCU\Final_DBC\20160113 RMS PM CAN DB.dbc  MsgList=M165_Motor_Position_Info  MsgName=M165_Motor_Position_Info  MsgIDType=Standard (11-bit identifier)  MsgIdentifier=165  MsgLength=8  SignalInfo=D1_Motor_Angle_Electrical$0$16$1$2$1$0$1.000000e-01$0$0$6.553500e+03$#D2_Motor_Speed$16$16$1$1$1$0$1$0$-32768$32767$#D3_Electrical_Output_Frequency$32$16$1$1$1$0$1.000000e-01$0$-3.276800e+03$3.276700e+03$#D4_Delta_Resolver_Filtered$48$16$1$1$1$0$1.000000e-01$0$-3.276800e+03$3.276700e+03$#  NSignals=4  StartBits=str2num('[int32(0);int32(16);int32(32);int32(48)]')  SignalSizes=str2num('[int32(16);int32(16);int32(16);int32(16)]')  ByteOrders=str2num('[int32(1);int32(1);int32(1);int32(1)]')  DataTypes=str2num('[int32(2);int32(1);int32(1);int32(1)]')  MultiplexTypes=str2num('[int32(1);int32(1);int32(1);int32(1)]')  MultiplexValues=str2num('[double(0);double(0);double(0);double(0)]')  Factors=str2num('[double(1.000000e-01);double(1);double(1.000000e-01);double(1.000000e-01)]')  Offsets=str2num('[double(0);double(0);double(0);double(0)]')  Minimums=str2num('[double(0);double(-32768);double(-3.276800e+03);double(-3.276800e+03)]')  Maximums=str2num('[double(6.553500e+03);double(32767);double(3.276700e+03);double(3.276700e+03)]')  Remote=off
      settings: DataFormat=CANdb specified signals
  Ground1 : Ground
  Rate Transition : RateTransition
  Out1 : Outport
  wires:
  Bus Selector1/1 -> Rate Transition/1  "<Motor_Speed>"
  CAN Pack1/1 -> Out1/1
  Ground1/1 -> CAN Pack1/1, CAN Pack1/3, CAN Pack1/4
  EM/1 -> Bus Selector1/1
  Rate Transition/1 -> CAN Pack1/2

== system EcoSIM3_P2_C2_WIP/Powertrain/Soft_ECUs_IO/VNT Vector/CANTx/EM/M170_Internal_States ==
  EM : Inport
  Bus Selector3 : BusSelector  OutputSignals=M170_Internal_States.VSM_State,M170_Internal_States.Inverter_Enable_Lockout,M170_Internal_States.Direction_Command_Feedback
  CAN Pack4 : canmsglib/CAN Pack  CANdbFile=C:\Users\EcoCAR_HIL\Documents\Khanna\EcoSIM3_P1_0_PHEV_TCU\Final_DBC\20160113 RMS PM CAN DB.dbc  MsgList=M170_Internal_States  MsgName=M170_Internal_States  MsgIDType=Standard (11-bit identifier)  MsgIdentifier=170  MsgLength=8  SignalInfo=D1_VSM_State$0$16$1$2$1$0$1$0$0$15$#D2_Inverter_State$16$8$1$2$1$0$1$0$0$255$#D3_Relay_1_Status$24$1$1$2$1$0$1$0$0$1$#D3_Relay_2_Status$25$1$1$2$1$0$1$0$0$1$#D3_Relay_3_Status$26$1$1$2$1$0$1$0$0$1$#D3_Relay_4_Status$27$1$1$2$1$0$1$0$0$1$#D3_Relay_5_Status$28$1$1$2$1$0$1$0$-Inf$Inf$#D3_Relay_6_Status$29$1$1$2$1$0$1$0$-Inf$Inf$#D4_Inverter_Discharge_State$37$3$1$2$1$0$1$0$0$7$#D4_Inverter_Run_Mode$32$1$1$2$1$0$1$0$0$1$#D5_Inverter_Command_Mode$40$1$1$2$1$0$1$0$0$1$#D6_Inverter_Enable_Lockout$55$1$1$2$1$0$1$0$0$1$#D6_Inverter_Enable_State$48$1$1$2$1$0$1$0$0$1$#D7_Direction_Command$56$8$1$2$1$0$1$0$0$1$#  NSignals=14  StartBits=str2num('[int32(0);int32(16);int32(24);int32(25);int32(26);int32(27);int32(28);int32(29);int32(37);int32(32);int32(40);int32(55);int32(48);int32(56)]')  SignalSizes=str2num('[int32(16);int32(8);int32(1);int32(1);int32(1);int32(1);int32(1);int32(1);int32(3);int32(1);int32(1);int32(1);int32(1);int32(8)]')  ByteOrders=str2num('[int32(1);int32(1);int32(1);int32(1);int32(1);int32(1);int32(1);int32(1);int32(1);int32(1);int32(1);int32(1);int32(1);int32(1)]')  DataTypes=str2num('[int32(2);int32(2);int32(2);int32(2);int32(2);int32(2);int32(2);int32(2);int32(2);int32(2);int32(2);int32(2);int32(2);int32(2)]')  MultiplexTypes=str2num('[int32(1);int32(1);int32(1);int32(1);int32(1);int32(1);int32(1);int32(1);int32(1);int32(1);int32(1);int32(1);int32(1);int32(1)]')  MultiplexValues=str2num('[double(0);double(0);double(0);double(0);double(0);double(0);double(0);double(0);double(0);double(0);double(0);double(0);double(0);double(0)]')  Factors=str2num('[double(1);double(1);double(1);double(1);double(1);double(1);double(1);double(1);double(1);double(1);double(1);double(1);double(1);double(1)]')  Offsets=str2num('[double(0);double(0);double(0);double(0);double(0);double(0);double(0);double(0);double(0);double(0);double(0);double(0);double(0);double(0)]')  Minimums=str2num('[double(0);double(0);double(0);double(0);double(0);double(0);double(-Inf);double(-Inf);double(0);double(0);double(0);double(0);double(0);double(0)]')  Maximums=str2num('[double(15);double(255);double(1);double(1);double(1);double(1);double(Inf);double(Inf);double(7);double(1);double(1);double(1);double(1);double(1)]')  Remote=off
      settings: DataFormat=CANdb specified signals
  Ground9 : Ground
  Rate Transition : RateTransition
  Rate Transition1 : RateTransition
  Rate Transition2 : RateTransition
  Out1 : Outport
  wires:
  Bus Selector3/2 -> Rate Transition1/1  "<Inverter_Enable_Lockout>"
  Bus Selector3/1 -> Rate Transition/1  "<VSM_State>"
  Ground9/1 -> CAN Pack4/13, CAN Pack4/11, CAN Pack4/10, CAN Pack4/9, CAN Pack4/8, CAN Pack4/7, CAN Pack4/6, CAN Pack4/5, CAN Pack4/4, CAN Pack4/3, CAN Pack4/2
  EM/1 -> Bus Selector3/1
  Rate Transition/1 -> CAN Pack4/1
  Rate Transition1/1 -> CAN Pack4/12
  CAN Pack4/1 -> Out1/1
  Bus Selector3/3 -> Rate Transition2/1  "<Direction_Command_Feedback>"
  Rate Transition2/1 -> CAN Pack4/14

== system EcoSIM3_P2_C2_WIP/Powertrain/Soft_ECUs_IO/VNT Vector/CANTx/EM/M171_Fault_Codes ==
  EM : Inport
  Bus Selector4 : BusSelector  OutputSignals=M171_Fault_Codes.POST_Fault,M171_Fault_Codes.RUN_Fault
  CAN Pack2 : canmsglib/CAN Pack  CANdbFile=C:\Users\EcoCAR_HIL\Documents\Khanna\EcoSIM3_P1_0_PHEV_TCU\Final_DBC\20160113 RMS PM CAN DB.dbc  MsgList=M171_Fault_Codes  MsgName=M171_Fault_Codes  MsgIDType=Standard (11-bit identifier)  MsgIdentifier=171  MsgLength=8  SignalInfo=D1_Post_Fault_Lo$0$16$1$2$1$0$1$0$0$65535$#D2_Post_Fault_Hi$16$16$1$2$1$0$1$0$0$65535$#D3_Run_Fault_Lo$32$16$1$2$1$0$1$0$0$65535$#D4_Run_Fault_Hi$48$16$1$2$1$0$1$0$0$65535$#  NSignals=4  StartBits=str2num('[int32(0);int32(16);int32(32);int32(48)]')  SignalSizes=str2num('[int32(16);int32(16);int32(16);int32(16)]')  ByteOrders=str2num('[int32(1);int32(1);int32(1);int32(1)]')  DataTypes=str2num('[int32(2);int32(2);int32(2);int32(2)]')  MultiplexTypes=str2num('[int32(1);int32(1);int32(1);int32(1)]')  MultiplexValues=str2num('[double(0);double(0);double(0);double(0)]')  Factors=str2num('[double(1);double(1);double(1);double(1)]')  Offsets=str2num('[double(0);double(0);double(0);double(0)]')  Minimums=str2num('[double(0);double(0);double(0);double(0)]')  Maximums=str2num('[double(65535);double(65535);double(65535);double(65535)]')  Remote=off
      settings: DataFormat=CANdb specified signals
  Ground2 : Ground
  Ground3 : Ground
  Rate Transition : RateTransition
  Rate Transition1 : RateTransition
  Out1 : Outport
  wires:
  Bus Selector4/2 -> Rate Transition1/1  "<RUN_Fault>"
  Bus Selector4/1 -> Rate Transition/1  "<POST_Fault>"
  Ground3/1 -> CAN Pack2/4
  Ground2/1 -> CAN Pack2/2
  EM/1 -> Bus Selector4/1
  Rate Transition/1 -> CAN Pack2/1
  Rate Transition1/1 -> CAN Pack2/3
  CAN Pack2/1 -> Out1/1

== system EcoSIM3_P2_C2_WIP/Powertrain/Soft_ECUs_IO/VNT Vector/CANTx/EM/M172_Torque_And_Timer_Info ==
  EM : Inport
  Bus Selector2 : BusSelector  OutputSignals=M172_Torque_And_Timer_Info.EM_Torque_Out_Nm
  CAN Pack8 : canmsglib/CAN Pack  CANdbFile=C:\Users\EcoCAR_HIL\Documents\Khanna\EcoSIM3_P1_0_PHEV_TCU\Final_DBC\20160113 RMS PM CAN DB.dbc  MsgList=M172_Torque_And_Timer_Info  MsgName=M172_Torque_And_Timer_Info  MsgIDType=Standard (11-bit identifier)  MsgIdentifier=172  MsgLength=8  SignalInfo=D1_Commanded_Torque$0$16$1$1$1$0$1.000000e-01$0$-3.276800e+03$3.276700e+03$#D2_Torque_Feedback$16$16$1$1$1$0$1.000000e-01$0$-3.276800e+03$3.276700e+03$#D3_Power_On_Timer$32$32$1$2$1$0$3.000000e-03$0$0$4294970000$#  NSignals=3  StartBits=str2num('[int32(0);int32(16);int32(32)]')  SignalSizes=str2num('[int32(16);int32(16);int32(32)]')  ByteOrders=str2num('[int32(1);int32(1);int32(1)]')  DataTypes=str2num('[int32(1);int32(1);int32(2)]')  MultiplexTypes=str2num('[int32(1);int32(1);int32(1)]')  MultiplexValues=str2num('[double(0);double(0);double(0)]')  Factors=str2num('[double(1.000000e-01);double(1.000000e-01);double(3.000000e-03)]')  Offsets=str2num('[double(0);double(0);double(0)]')  Minimums=str2num('[double(-3.276800e+03);double(-3.276800e+03);double(0)]')  Maximums=str2num('[double(3.276700e+03);double(3.276700e+03);double(4294970000)]')  Remote=off
      settings: DataFormat=CANdb specified signals
  Ground4 : Ground
  Rate Transition : RateTransition
  Out1 : Outport
  wires:
  Bus Selector2/1 -> Rate Transition/1  "<EM_Torque_Out_Nm>"
  EM/1 -> Bus Selector2/1
  Ground4/1 -> CAN Pack8/1, CAN Pack8/3
  CAN Pack8/1 -> Out1/1
  Rate Transition/1 -> CAN Pack8/2

== system EcoSIM3_P2_C2_WIP/Powertrain/Soft_ECUs_IO/VNT Vector/CANTx/ESS/BCM_Data ==
  ESS : Inport
  Bus Selector1 : BusSelector  OutputSignals=BCM_Data1.bcm_cell_tmax,BCM_Data1.bcm_cell_tmin,BCM_Data1.bcm_veh_mon
  CAN Pack6 : canmsglib/CAN Pack  CANdbFile=C:\Users\EcoCAR_HIL\Documents\Khanna\EcoSIM3_P1_0_PHEV_TCU\Final_DBC\BCM_VehBus_Std.dbc  MsgList=BCM_Data1  MsgName=BCM_Data1  MsgIDType=Standard (11-bit identifier)  MsgIdentifier=1072  MsgLength=8  SignalInfo=bcm_cell_tmax$32$8$2$2$1$0$5.000000e-01$-40$-40$85$#bcm_cell_tmin$40$8$2$2$1$0$5.000000e-01$-40$-40$85$#bcm_cell_vmax$8$13$2$2$1$0$1.000000e-03$0$0$5$#bcm_cell_vmin$24$13$2$2$1$0$1.000000e-03$0$0$5$#bcm_chga_ena$7$1$2$2$1$0$1$0$0$1$#bcm_chga_mon$22$1$2$2$1$0$1$0$0$1$#bcm_lvbat$56$8$2$2$1$0$1.000000e-01$0$0$25$#bcm_mod_ena$23$1$2$2$1$0$1$0$0$1$#bcm_veh_mon$21$1$2$2$1$0$1$0$0$1$#  NSignals=9  StartBits=str2num('[int32(32);int32(40);int32(8);int32(24);int32(7);int32(22);int32(56);int32(23);int32(21)]')  SignalSizes=str2num('[int32(8);int32(8);int32(13);int32(13);int32(1);int32(1);int32(8);int32(1);int32(1)]')  ByteOrders=str2num('[int32(2);int32(2);int32(2);int32(2);int32(2);int32(2);int32(2);int32(2);int32(2)]')  DataTypes=str2num('[int32(2);int32(2);int32(2);int32(2);int32(2);int32(2);int32(2);int32(2);int32(2)]')  MultiplexTypes=str2num('[int32(1);int32(1);int32(1);int32(1);int32(1);int32(1);int32(1);int32(1);int32(1)]')  MultiplexValues=str2num('[double(0);double(0);double(0);double(0);double(0);double(0);double(0);double(0);double(0)]')  Factors=str2num('[double(5.000000e-01);double(5.000000e-01);double(1.000000e-03);double(1.000000e-03);double(1);double(1);double(1.000000e-01);double(1);double(1)]')  Offsets=str2num('[double(-40);double(-40);double(0);double(0);double(0);double(0);double(0);double(0);double(0)]')  Minimums=str2num('[double(-40);double(-40);double(0);double(0);double(0);double(0);double(0);double(0);double(0)]')  Maximums=str2num('[double(85);double(85);double(5);double(5);double(1);double(1);double(25);double(1);double(1)]')  Remote=off
      settings: DataFormat=CANdb specified signals
  CAN Transmit6 : canlib/CAN Transmit  BlockHandle=11914.0001  DeviceMenu=Vector Virtual 1 (Channel 1)  Device=Vector Virtual 1 (Channel 1)  ObjConstructor=canChannel('Vector', 'Virtual 1', 1)  EnablePeriodicTransmit=off  MessagePeriod=1.000
  Ground{14..19} (6 alike) : Ground
  Rate Transition : RateTransition
  Rate Transition1 : RateTransition
  Rate Transition2 : RateTransition
  wires:
  Ground15/1 -> CAN Pack6/4
  Bus Selector1/2 -> Rate Transition1/1  "<bcm_cell_tmin>"
  Ground16/1 -> CAN Pack6/5
  Ground19/1 -> CAN Pack6/8
  Ground17/1 -> CAN Pack6/6
  Ground18/1 -> CAN Pack6/7
  Ground14/1 -> CAN Pack6/3
  Bus Selector1/3 -> Rate Transition2/1  "<bcm_veh_mon>"
  Bus Selector1/1 -> Rate Transition/1  "<bcm_cell_tmax>"
  ESS/1 -> Bus Selector1/1
  Rate Transition/1 -> CAN Pack6/1
  Rate Transition1/1 -> CAN Pack6/2
  Rate Transition2/1 -> CAN Pack6/9
  CAN Pack6/1 -> CAN Transmit6/1

== system EcoSIM3_P2_C2_WIP/Powertrain/Soft_ECUs_IO/VNT Vector/CANTx/ESS/BCM_Limits ==
  ESS : Inport
  Bus Selector1 : BusSelector  OutputSignals=BCM_Limits.bcm_chg_buf,BCM_Limits.bcm_dis_buf
  CAN Pack1 : canmsglib/CAN Pack  CANdbFile=C:\Users\EcoCAR_HIL\Documents\Khanna\EcoSIM3_P1_0_PHEV_TCU\Final_DBC\BCM_VehBus_Std.dbc  MsgList=BCM_Limits  MsgName=BCM_Limits  MsgIDType=Standard (11-bit identifier)  MsgIdentifier=1056  MsgLength=8  SignalInfo=bcm_cell_overvolt$55$1$2$2$1$0$1$0$0$1$#bcm_cell_undervolt$54$1$2$2$1$0$1$0$0$1$#bcm_chg_buf$32$8$2$2$1$0$5.000000e-01$0$0$100$#bcm_chg_max$16$12$2$2$1$0$2.500000e-01$0$0$1000$#bcm_dis_buf$24$8$2$2$1$0$5.000000e-01$0$0$100$#bcm_dis_max$12$12$2$2$1$0$2.500000e-01$0$0$1000$#bcm_t_coolant$40$8$2$2$1$0$5.000000e-01$-40$-40$85$#  NSignals=7  StartBits=str2num('[int32(55);int32(54);int32(32);int32(16);int32(24);int32(12);int32(40)]')  SignalSizes=str2num('[int32(1);int32(1);int32(8);int32(12);int32(8);int32(12);int32(8)]')  ByteOrders=str2num('[int32(2);int32(2);int32(2);int32(2);int32(2);int32(2);int32(2)]')  DataTypes=str2num('[int32(2);int32(2);int32(2);int32(2);int32(2);int32(2);int32(2)]')  MultiplexTypes=str2num('[int32(1);int32(1);int32(1);int32(1);int32(1);int32(1);int32(1)]')  MultiplexValues=str2num('[double(0);double(0);double(0);double(0);double(0);double(0);double(0)]')  Factors=str2num('[double(1);double(1);double(5.000000e-01);double(2.500000e-01);double(5.000000e-01);double(2.500000e-01);double(5.000000e-01)]')  Offsets=str2num('[double(0);double(0);double(0);double(0);double(0);double(0);double(-40)]')  Minimums=str2num('[double(0);double(0);double(0);double(0);double(0);double(0);double(-40)]')  Maximums=str2num('[double(1);double(1);double(100);double(1000);double(100);double(1000);double(85)]')  Remote=off
      settings: DataFormat=CANdb specified signals
  CAN Transmit6 : canlib/CAN Transmit  BlockHandle=11942.0001  DeviceMenu=Vector Virtual 1 (Channel 1)  Device=Vector Virtual 1 (Channel 1)  ObjConstructor=canChannel('Vector', 'Virtual 1', 1)  EnablePeriodicTransmit=off  MessagePeriod=1.000
  Ground{4,6..9} (5 alike) : Ground
  Rate Transition : RateTransition
  Rate Transition1 : RateTransition
  wires:
  Ground8/1 -> CAN Pack1/6
  Ground4/1 -> CAN Pack1/1
  Ground9/1 -> CAN Pack1/7
  Ground7/1 -> CAN Pack1/4
  Ground6/1 -> CAN Pack1/2
  Bus Selector1/1 -> Rate Transition/1  "<bcm_chg_buf>"
  ESS/1 -> Bus Selector1/1
  Bus Selector1/2 -> Rate Transition1/1  "<bcm_dis_buf>"
  Rate Transition/1 -> CAN Pack1/3
  Rate Transition1/1 -> CAN Pack1/5
  CAN Pack1/1 -> CAN Transmit6/1
